simulink model "Basics_Simulink"  (R2024b)
settings: Solver=VariableStepAuto  StartTime=0.0  StopTime=10.0  RelTol=1e-3
settings Model: Creator=abdal  LastModifiedBy=abdal

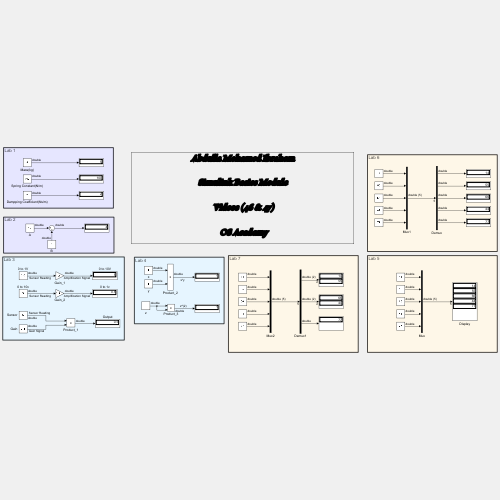
[thumbnail: Simulink's stored preview of the top-level diagram]
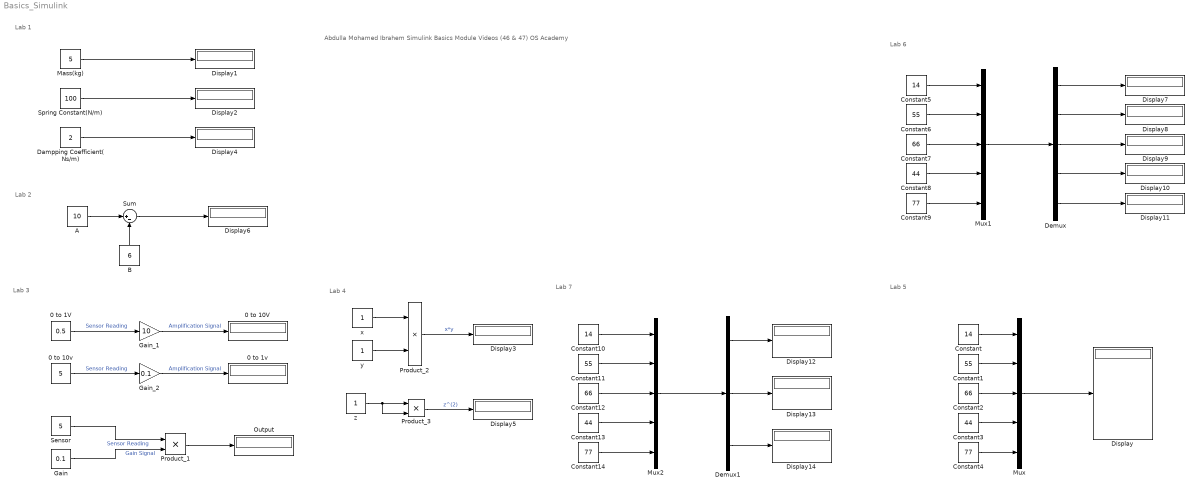
== system Basics_Simulink ==
  note: Abdulla Mohamed Ibrahem
      | Simulink Basics Module
      | Videos (46 & 47)
      | OS Academy
  note: Lab 7
  note: Lab 4
  note: Lab 3
  note: Lab 2
  note: Lab 1
  note: Lab 6
  note: Lab 5
  0 to 10V : Display
  0 to 10v : Constant  Value=5
  0 to 1V : Constant  Value=0.5
  0 to 1v : Display
  A : Constant  Value=10
  B : Constant  Value=6
  Constant : Constant  Value=14
  Constant1 : Constant  Value=55
  Constant10 : Constant  Value=14
  Constant11 : Constant  Value=55
  Constant12 : Constant  Value=66
  Constant13 : Constant  Value=44
  Constant14 : Constant  Value=77
  Constant2 : Constant  Value=66
  Constant3 : Constant  Value=44
  Constant4 : Constant  Value=77
  Constant5 : Constant  Value=14
  Constant6 : Constant  Value=55
  Constant7 : Constant  Value=66
  Constant8 : Constant  Value=44
  Constant9 : Constant  Value=77
  Dampping Coefficient(Ns/m) : Constant  Value=2
  Demux : Demux  Outputs=5
  Demux1 : Demux  Outputs=3
  Display{,1..14} (15 alike) : Display
  Gain : Constant  Value=0.1
  Gain_1 : Gain  Gain=10
  Gain_2 : Gain  Gain=0.1
  Mass(kg) : Constant  Value=5
  Mux : Mux  Inputs=5
  Mux1 : Mux  Inputs=5
  Mux2 : Mux  Inputs=5
  Output : Display
  Product_1 : Product
  Product_2 : Product
  Product_3 : Product
  Sensor : Constant  Value=5
  Spring Constant(N/m) : Constant  Value=100
  Sum : Sum  Inputs=|+-
  x : Constant
  y : Constant
  z : Constant
  wires:
  Dampping Coefficient(Ns/m)/1 -> Display4/1
  Spring Constant(N/m)/1 -> Display2/1
  Mass(kg)/1 -> Display1/1
  A/1 -> Sum/1
  B/1 -> Sum/2
  Sum/1 -> Display6/1
  0 to 1V/1 -> Gain_1/1  "Sensor Reading"
  Gain_1/1 -> 0 to 10V/1  "Amplification Signal"
  Gain_2/1 -> 0 to 1v/1  "Amplification Signal"
  0 to 10v/1 -> Gain_2/1  "Sensor Reading"
  Sensor/1 -> Product_1/1  "Sensor Reading"
  Gain/1 -> Product_1/2  "Gain Signal"
  Product_1/1 -> Output/1
  x/1 -> Product_2/1
  y/1 -> Product_2/2
  Product_2/1 -> Display3/1  "x*y"
  z/1 -> Product_3/2, Product_3/1
  Product_3/1 -> Display5/1  "z^(2)"
  Constant/1 -> Mux/1
  Constant1/1 -> Mux/2
  Constant2/1 -> Mux/3
  Constant3/1 -> Mux/4
  Constant4/1 -> Mux/5
  Mux/1 -> Display/1
  Mux1/1 -> Demux/1
  Constant9/1 -> Mux1/5
  Constant8/1 -> Mux1/4
  Constant7/1 -> Mux1/3
  Constant6/1 -> Mux1/2
  Constant5/1 -> Mux1/1
  Demux/1 -> Display7/1
  Demux/2 -> Display8/1
  Demux/3 -> Display9/1
  Demux/4 -> Display10/1
  Demux/5 -> Display11/1
  Constant10/1 -> Mux2/1
  Constant11/1 -> Mux2/2
  Constant12/1 -> Mux2/3
  Constant13/1 -> Mux2/4
  Constant14/1 -> Mux2/5
  Mux2/1 -> Demux1/1
  Demux1/1 -> Display12/1
  Demux1/2 -> Display13/1
  Demux1/3 -> Display14/1
